simulink model "FF_Jan24_Pool_Test"  (R2025b)
settings: Solver=FixedStepAuto  StartTime=0.0  StopTime=inf  FixedStep=dt_sim  RelTol=rel_tol  AbsTol=abs_tol
undefined symbols (not defined in the file or in its folder): enable_publish_flag, mission_file
libraries: ros2lib x1
settings Model: Creator=koryh  LastModifiedBy=cyclone

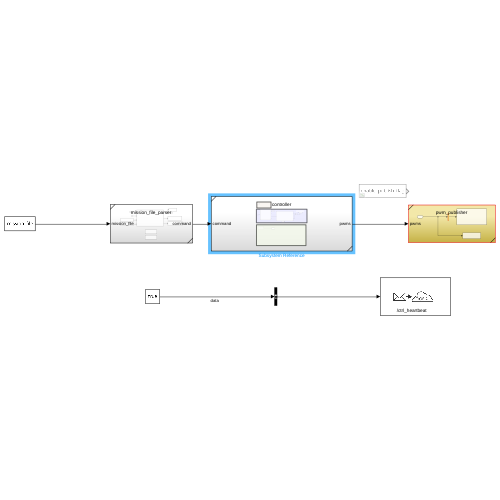
[thumbnail: Simulink's stored preview of the top-level diagram]
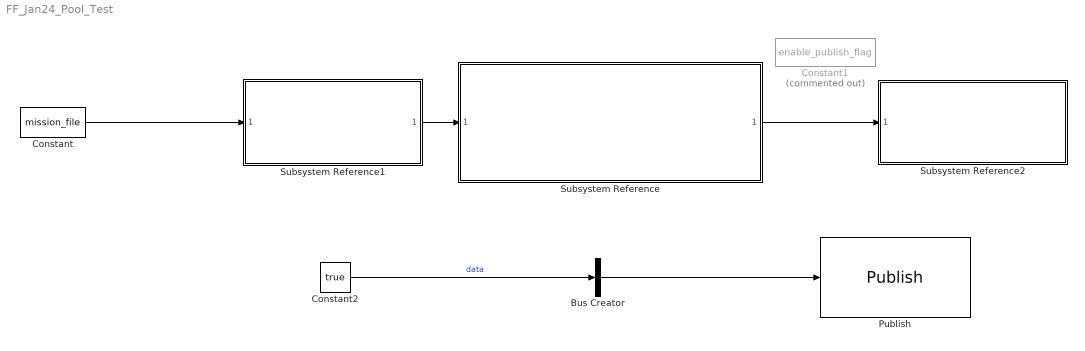
== system FF_Jan24_Pool_Test ==
  Bus Creator : BusCreator  Inputs=1  OutDataTypeStr=Bus: SL_Bus_std_msgs_Bool  NonVirtualBus=on
  Constant : Constant  Value=mission_file
  Constant1 : Constant  Commented=on  Value=enable_publish_flag
  Constant2 : Constant  Value=true  OutDataTypeStr=boolean
  Publish : ros2lib/Publish  topicSource=Specify your own  topic=/ctrl_heartbeat  messageType=std_msgs/Bool  QOSHistory=Keep last  QOSDepth=10  QOSReliability=Reliable  QOSDurability=Volatile  QOSDeadline=Inf  QOSLifespan=Inf  QOSLiveliness=Automatic  QOSLeaseDuration=Inf  QOSAvoidROSNamespaceConventions=off
  Subsystem Reference : Subsystem  ReferencedSubsystem=controller
  Subsystem Reference1 : Subsystem  ReferencedSubsystem=mission_file_parser
  Subsystem Reference2 : Subsystem  ReferencedSubsystem=pwm_publisher
  wires:
  Subsystem Reference1/1 -> Subsystem Reference/1
  Constant/1 -> Subsystem Reference1/1
  Subsystem Reference/1 -> Subsystem Reference2/1
  Constant2/1 -> Bus Creator/1  "data"
  Bus Creator/1 -> Publish/1
